simulink model "PX4HITLConnector"  (R2026a)
settings: Solver=VariableStepAuto
values from neighbouring files (symbols this model uses):
  gpsFreq = 25    [setUpHITLConnection.m]
  heartbeatFreq = 1    [setUpHITLConnection.m]
  SampleTime = 0.008    [setUpHITLConnection.m]
undefined symbols (not defined in the file or in its folder): controllerArmed, EngineCommandBus, Payload, ServosCommandBus
libraries: uavmavlinklib x7, simulink x4, px4MAVLinkBridgelib x2
settings Model: Creator=Usuario  LastModifiedBy=Usuario

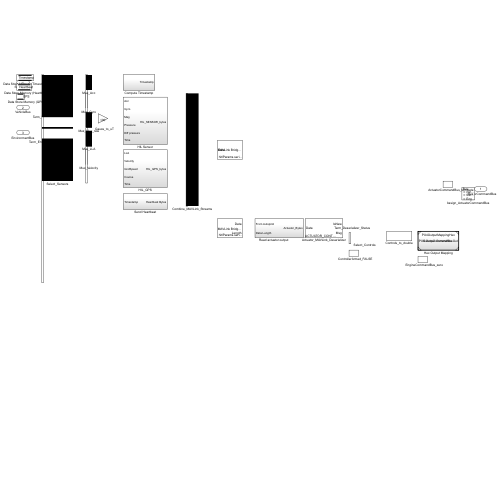
[thumbnail: Simulink's stored preview of the top-level diagram]
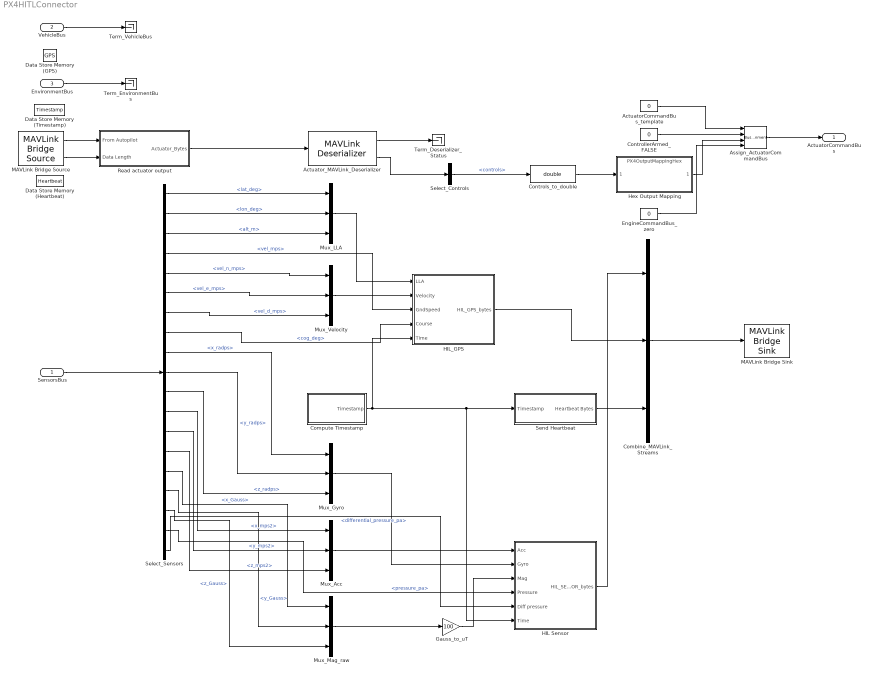
== system PX4HITLConnector ==
  SensorsBus : Inport  OutDataTypeStr=Bus: SensorsBus
  VehicleBus : Inport  Port=2  OutDataTypeStr=Bus: VehicleBus
  EnvironmentBus : Inport  Port=3  OutDataTypeStr=Bus: EnvironmentBus
  ActuatorCommandBus_template : Constant  Value=0  OutDataTypeStr=Bus: ActuatorCommandBus
  Actuator_MAVLink_Deserializer : uavmavlinklib/MAVLink Deserializer  dialectSource=Select from standard MAVLink dialects  dialect=common.xml  dialectCustom=common.xml  version=2  messageType=HIL_ACTUATOR_CONTROLS  inputDataLength=off  SystemIDFilter=off  systemID=1  ComponentIDFilter=off  componentID=1  queueMsg=off  queueMsgSize=50  dropNum=off
  Assign_ActuatorCommandBus : BusAssignment  AssignedSignals=controllerArmed,ServosCommandBus,EngineCommandBus
  Combine_MAVLink_Streams : Mux  Inputs=3
  Compute Timestamp : Subsystem  Priority=1
  ControllerArmed_FALSE : Constant  Value=0  OutDataTypeStr=double
  Controls_to_double : DataTypeConversion  OutDataTypeStr=double  SaturateOnIntegerOverflow=off  RndMeth=Floor
  Data Store Memory (GPS) : DataStoreMemory  DataStoreName=GPS  WriteAfterWriteMsg=warning  ShowAdditionalParam=off
  Data Store Memory (Heartbeat) : DataStoreMemory  DataStoreName=Heartbeat  WriteAfterWriteMsg=warning  ShowAdditionalParam=off
  Data Store Memory (Timestamp) : DataStoreMemory  DataStoreName=Timestamp  WriteAfterWriteMsg=warning  ShowAdditionalParam=off
  EngineCommandBus_zero : Constant  Value=0  OutDataTypeStr=Bus: EngineCommandBus
  Gauss_to_uT : Gain  Gain=100
  HIL Sensor : Subsystem  Priority=2
  HIL_GPS : Subsystem  Priority=3
  Hex Output Mapping : ModelReference  ModelNameDialog=PX4OutputMappingHex.slx  SimulationMode=Normal  ModelReferenceVersion=1.15
  MAVLink Bridge Sink : px4MAVLinkBridgelib/MAVLink Bridge Sink  PixhawkSerialPorttemp=Specify manually  PixhawkSerialPortManually=hitlParams.serialPort  FieldTable={'UDP', '127.0.0.1', '14550'}
  MAVLink Bridge Source : px4MAVLinkBridgelib/MAVLink Bridge Source  PixhawkSerialPorttemp=Specify manually  PixhawkSerialPortManually=hitlParams.serialPort  dataLength=1024  FieldTable={'UDP', '127.0.0.1', '14550'}  SampleTime=SampleTime
  Mux_Acc : Mux  Inputs=3
  Mux_Gyro : Mux  Inputs=3
  Mux_LLA : Mux  Inputs=3
  Mux_Mag_raw : Mux  Inputs=3
  Mux_Velocity : Mux  Inputs=3
  Read actuator output : Subsystem
  Select_Controls : BusSelector  OutputSignals=Payload.controls
  Select_Sensors : BusSelector  OutputSignals=GPSSensorBus.lat_deg,GPSSensorBus.lon_deg,GPSSensorBus.alt_m,GPSSensorBus.vel_mps,GPSSensorBus.vel_n_mps,GPSSensorBus.vel_e_mps,GPSSensorBus.vel_d_mps,GPSSensorBus.cog_deg,INSSensorBus.GyroSensorBus.x_radps,INSSensorBus.GyroSensorBus.y_radps,INSSensorBus.GyroSensorBus.z_radps,INSSensorBus.AccelSensorBus.x_mps2,INSSensorBus.AccelSensorBus.y_mps2,INSSensorBus.AccelSensorBus.z_mps2,INSSensorBus.MagSensorBus.x_Gauss,INSSensorBus.MagSensorBus.y_Gauss,INSSensorBus.MagSensorBus.z_Gauss,ADCSensorBus.BaroSensorBus.pressure_pa,ADCSensorBus.DiffPressureSensorBus.differential_pressure_pa
  Send Heartbeat : Subsystem  Priority=4
  Term_Deserializer_Status : Terminator
  Term_EnvironmentBus : Terminator
  Term_VehicleBus : Terminator
  ActuatorCommandBus : Outport  OutDataTypeStr=Bus: ActuatorCommandBus
  wires:
  Select_Sensors/18 -> HIL Sensor/4(Pressure)  "<pressure_pa>"
  Select_Sensors/1 -> Mux_LLA/1  "<lat_deg>"
  HIL_GPS/1(HIL_GPS_bytes) -> Combine_MAVLink_Streams/2
  Actuator_MAVLink_Deserializer/1 -> Term_Deserializer_Status/1
  VehicleBus/1 -> Term_VehicleBus/1
  MAVLink Bridge Source/2 -> Read actuator output/2(Data Length)
  Read actuator output/1(Actuator_Bytes) -> Actuator_MAVLink_Deserializer/1
  Mux_Mag_raw/1 -> Gauss_to_uT/1
  SensorsBus/1 -> Select_Sensors/1
  EnvironmentBus/1 -> Term_EnvironmentBus/1
  MAVLink Bridge Source/1 -> Read actuator output/1(From Autopilot)
  Select_Sensors/2 -> Mux_LLA/2  "<lon_deg>"
  Mux_Acc/1 -> HIL Sensor/1(Acc)
  Select_Sensors/3 -> Mux_LLA/3  "<alt_m>"
  Mux_Gyro/1 -> HIL Sensor/2(Gyro)
  Actuator_MAVLink_Deserializer/2 -> Select_Controls/1
  Select_Sensors/4 -> HIL_GPS/3(GndSpeed)  "<vel_mps>"
  Select_Sensors/5 -> Mux_Velocity/1  "<vel_n_mps>"
  Select_Sensors/11 -> Mux_Gyro/3  "<z_radps>"
  Select_Sensors/6 -> Mux_Velocity/2  "<vel_e_mps>"
  Select_Sensors/7 -> Mux_Velocity/3  "<vel_d_mps>"
  Mux_Velocity/1 -> HIL_GPS/2(Velocity)
  Select_Sensors/8 -> HIL_GPS/4(Course)  "<cog_deg>"
  HIL Sensor/1(HIL_SENSOR_bytes) -> Combine_MAVLink_Streams/1
  Select_Sensors/9 -> Mux_Gyro/1  "<x_radps>"
  ActuatorCommandBus_template/1 -> Assign_ActuatorCommandBus/1
  Select_Sensors/10 -> Mux_Gyro/2  "<y_radps>"
  Select_Sensors/12 -> Mux_Acc/1  "<x_mps2>"
  Select_Sensors/13 -> Mux_Acc/2  "<y_mps2>"
  Select_Sensors/14 -> Mux_Acc/3  "<z_mps2>"
  Select_Sensors/15 -> Mux_Mag_raw/1  "<x_Gauss>"
  Select_Sensors/16 -> Mux_Mag_raw/2  "<y_Gauss>"
  Select_Sensors/17 -> Mux_Mag_raw/3  "<z_Gauss>"
  Select_Sensors/19 -> HIL Sensor/5(Diff pressure)  "<differential_pressure_pa>"
  Mux_LLA/1 -> HIL_GPS/1(LLA)
  Compute Timestamp/1(Timestamp) -> Send Heartbeat/1(Timestamp), HIL Sensor/6(Time), HIL_GPS/5(Time)
  Controls_to_double/1 -> Hex Output Mapping/1
  Select_Controls/1 -> Controls_to_double/1  "<controls>"
  Gauss_to_uT/1 -> HIL Sensor/3(Mag)
  Combine_MAVLink_Streams/1 -> MAVLink Bridge Sink/1
  Send Heartbeat/1(Heartbeat Bytes) -> Combine_MAVLink_Streams/3
  ControllerArmed_FALSE/1 -> Assign_ActuatorCommandBus/2
  Hex Output Mapping/1 -> Assign_ActuatorCommandBus/3
  EngineCommandBus_zero/1 -> Assign_ActuatorCommandBus/4
  Assign_ActuatorCommandBus/1 -> ActuatorCommandBus/1

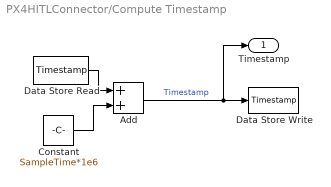
== system PX4HITLConnector/Compute Timestamp ==
  Add : Sum
  Constant : Constant  Value=SampleTime*1e6  OutDataTypeStr=uint64  SampleTime=SampleTime
  Data Store Read : DataStoreRead  DataStoreName=Timestamp  SampleTime=SampleTime  IndexOptions=Index vector (dialog)  Indices=1  OutputSizes=1
  Data Store Write : DataStoreWrite  DataStoreName=Timestamp  SampleTime=SampleTime  IndexOptions=Index vector (dialog)  Indices=1  OutputSizes=1
  Timestamp : Outport
  wires:
  Constant/1 -> Add/2
  Add/1 -> Data Store Write/1, Timestamp/1  "Timestamp"
  Data Store Read/1 -> Add/1

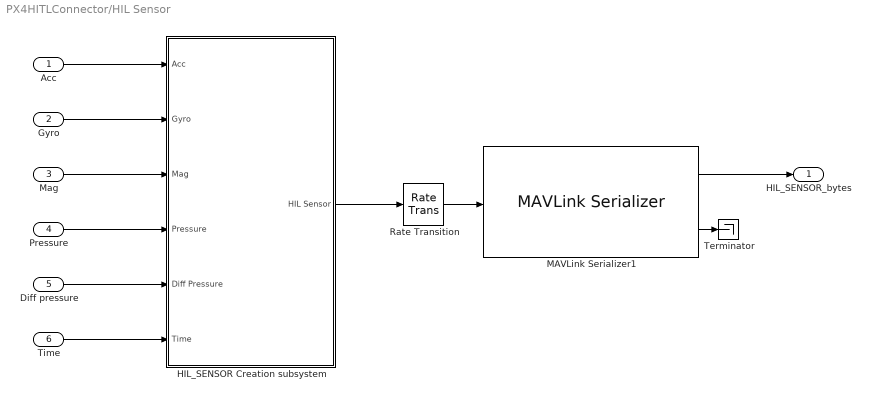
== system PX4HITLConnector/HIL Sensor ==
  Acc : Inport
  Gyro : Inport  Port=2
  Mag : Inport  Port=3
  Pressure : Inport  Port=4
  Diff pressure : Inport  Port=5
  Time : Inport  Port=6
  HIL_SENSOR Creation subsystem : Subsystem
  MAVLink Serializer1 : uavmavlinklib/MAVLink Serializer  dialectSource=Select from standard MAVLink dialects  dialect=common.xml  dialectCustom=common.xml  version=2  messageType=HIL_SENSOR
  Rate Transition : RateTransition  OutPortSampleTime=SampleTime
  Terminator : Terminator
  HIL_SENSOR_bytes : Outport
  wires:
  Time/1 -> HIL_SENSOR Creation subsystem/6(Time)
  HIL_SENSOR Creation subsystem/1(HIL Sensor) -> Rate Transition/1
  MAVLink Serializer1/1 -> HIL_SENSOR_bytes/1
  MAVLink Serializer1/2 -> Terminator/1
  Rate Transition/1 -> MAVLink Serializer1/1
  Diff pressure/1 -> HIL_SENSOR Creation subsystem/5(Diff Pressure)
  Pressure/1 -> HIL_SENSOR Creation subsystem/4(Pressure)
  Mag/1 -> HIL_SENSOR Creation subsystem/3(Mag)
  Gyro/1 -> HIL_SENSOR Creation subsystem/2(Gyro)
  Acc/1 -> HIL_SENSOR Creation subsystem/1(Acc)

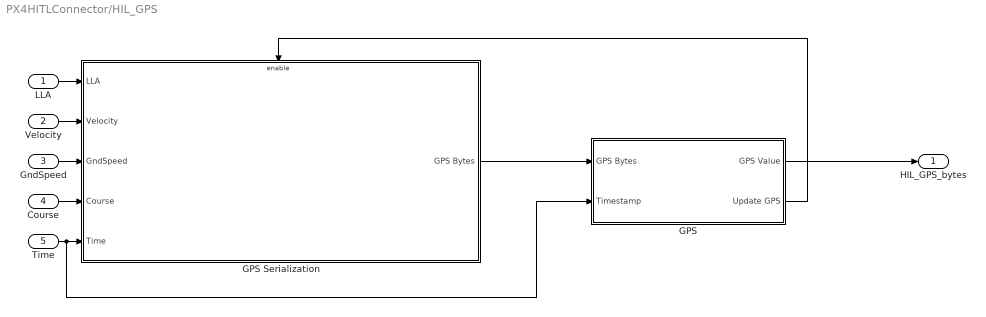
== system PX4HITLConnector/HIL_GPS ==
  LLA : Inport
  Velocity : Inport  Port=2
  GndSpeed : Inport  Port=3
  Course : Inport  Port=4
  Time : Inport  Port=5
  GPS : Subsystem
  GPS Serialization : Subsystem
  HIL_GPS_bytes : Outport
  wires:
  GPS/2(Update GPS) -> GPS Serialization/Enable
  GPS/1(GPS Value) -> HIL_GPS_bytes/1
  GPS Serialization/1(GPS Bytes) -> GPS/1(GPS Bytes)
  Time/1 -> GPS Serialization/5(Time), GPS/2(Timestamp)
  Course/1 -> GPS Serialization/4(Course)
  GndSpeed/1 -> GPS Serialization/3(GndSpeed)
  Velocity/1 -> GPS Serialization/2(Velocity)
  LLA/1 -> GPS Serialization/1(LLA)

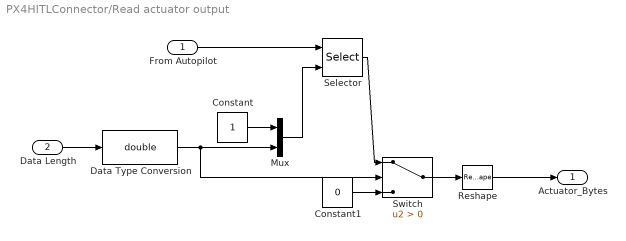
== system PX4HITLConnector/Read actuator output ==
  From Autopilot : Inport
  Data Length : Inport  Port=2
  Constant : Constant  SampleTime=SampleTime
  Constant1 : Constant  Value=0  OutDataTypeStr=uint8  SampleTime=SampleTime
  Data Type Conversion : DataTypeConversion  OutDataTypeStr=double  SaturateOnIntegerOverflow=off  RndMeth=Floor
  Mux : Mux  Inputs=2
  Reshape : Reshape
  Selector : Selector  InputPortWidth=MAVLink_Input_Read_Size  IndexOptions=Starting and ending indices (port)  Indices=[1 3]  OutputSizes=1
  Switch : Switch  Criteria=u2 > Threshold  SaturateOnIntegerOverflow=off  InputSameDT=off
  Actuator_Bytes : Outport
  wires:
  Constant1/1 -> Switch/3
  Reshape/1 -> Actuator_Bytes/1
  Data Type Conversion/1 -> Mux/2, Switch/2
  Selector/1 -> Switch/1
  Switch/1 -> Reshape/1
  From Autopilot/1 -> Selector/1
  Data Length/1 -> Data Type Conversion/1
  Constant/1 -> Mux/1
  Mux/1 -> Selector/2

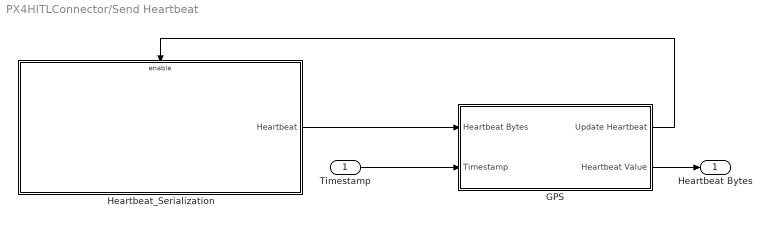
== system PX4HITLConnector/Send Heartbeat ==
  Timestamp : Inport
  GPS : Subsystem
  Heartbeat_Serialization : Subsystem
  Heartbeat Bytes : Outport
  wires:
  GPS/2(Heartbeat Value) -> Heartbeat Bytes/1
  GPS/1(Update Heartbeat) -> Heartbeat_Serialization/Enable
  Timestamp/1 -> GPS/2(Timestamp)
  Heartbeat_Serialization/1(Heartbeat) -> GPS/1(Heartbeat Bytes)

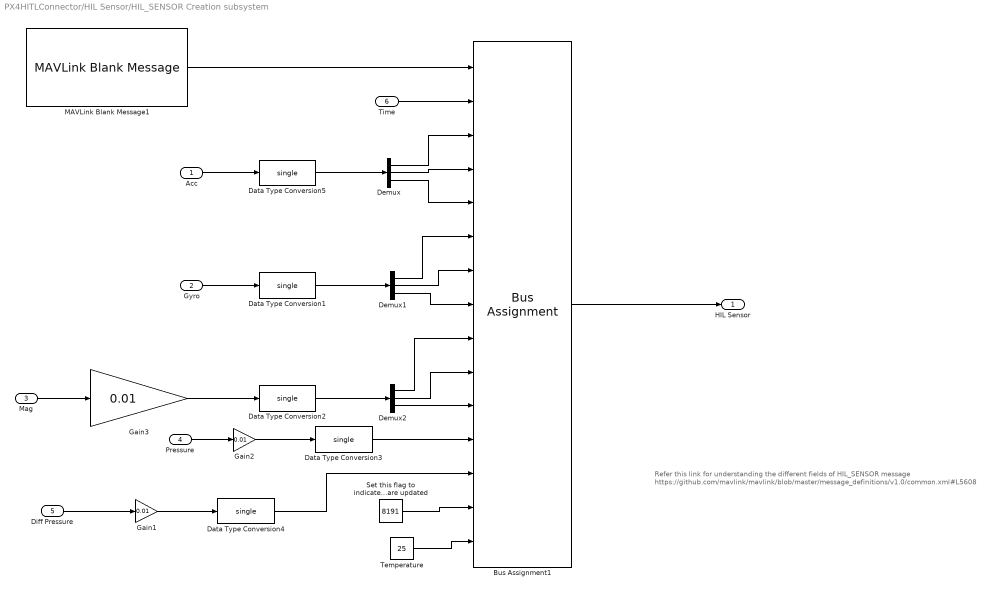
== system PX4HITLConnector/HIL Sensor/HIL_SENSOR Creation subsystem ==
  note: Refer this link for understanding the different fields of HIL_SENSOR message https://github.com/mavlink/mavlink/blob/master/message_definitions/v1.0/common.xml#L5608
  Acc : Inport
  Gyro : Inport  Port=2
  Mag : Inport  Port=3
  Pressure : Inport  Port=4
  Diff Pressure : Inport  Port=5
  Time : Inport  Port=6
  Bus Assignment1 : BusAssignment  AssignedSignals=Payload.time_usec,Payload.xacc,Payload.yacc,Payload.zacc,Payload.xgyro,Payload.ygyro,Payload.zgyro,Payload.xmag,Payload.ymag,Payload.zmag,Payload.abs_pressure,Payload.diff_pressure,Payload.fields_updated,Payload.temperature
  Data Type Conversion{1..5} (5 alike) : DataTypeConversion  OutDataTypeStr=single  SaturateOnIntegerOverflow=off  RndMeth=Floor
  Demux : Demux  Outputs=3
  Demux1 : Demux  Outputs=3
  Demux2 : Demux  Outputs=3
  Gain1 : Gain  Gain=0.01  OutDataTypeStr=single
  Gain2 : Gain  Gain=0.01  OutDataTypeStr=single
  Gain3 : Gain  Gain=0.01
  MAVLink Blank Message1 : uavmavlinklib/MAVLink Blank Message  dialectSource=Select from standard MAVLink dialects  dialect=common.xml  dialectCustom=common.xml  version=2  messageType=HIL_SENSOR  SystemID=2  ComponentID=51  SampleTime=-1
  Set this flag to indicate all flags are updated : Constant  Value=8191  OutDataTypeStr=Inherit: Inherit via back propagation  SampleTime=-1
  Temperature : Constant  Value=25  OutDataTypeStr=Inherit: Inherit via back propagation  SampleTime=-1
  HIL Sensor : Outport
  wires:
  Data Type Conversion4/1 -> Bus Assignment1/13
  Gain1/1 -> Data Type Conversion4/1
  Diff Pressure/1 -> Gain1/1
  Temperature/1 -> Bus Assignment1/15
  Gain2/1 -> Data Type Conversion3/1
  Time/1 -> Bus Assignment1/2
  Pressure/1 -> Gain2/1
  Set this flag to indicate all flags are updated/1 -> Bus Assignment1/14
  Gain3/1 -> Data Type Conversion2/1
  Data Type Conversion3/1 -> Bus Assignment1/12
  Acc/1 -> Data Type Conversion5/1
  Demux1/2 -> Bus Assignment1/7
  Demux/2 -> Bus Assignment1/4
  Demux2/1 -> Bus Assignment1/9
  MAVLink Blank Message1/1 -> Bus Assignment1/1
  Demux/1 -> Bus Assignment1/3
  Data Type Conversion5/1 -> Demux/1
  Demux2/3 -> Bus Assignment1/11
  Demux2/2 -> Bus Assignment1/10
  Demux/3 -> Bus Assignment1/5
  Bus Assignment1/1 -> HIL Sensor/1
  Gyro/1 -> Data Type Conversion1/1
  Data Type Conversion1/1 -> Demux1/1
  Demux1/3 -> Bus Assignment1/8
  Mag/1 -> Gain3/1
  Demux1/1 -> Bus Assignment1/6
  Data Type Conversion2/1 -> Demux2/1

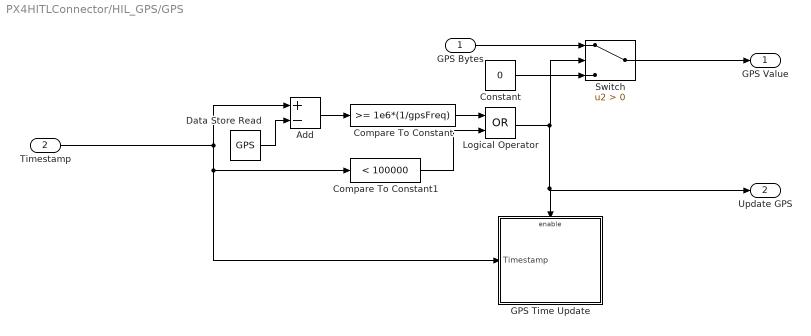
== system PX4HITLConnector/HIL_GPS/GPS ==
  GPS Bytes : Inport
  Timestamp : Inport  Port=2
  Add : Sum  Inputs=+-
  Compare To Constant : simulink/Logic and Bit Operations/Compare To Constant  relop=>=  const=1e6*(1/gpsFreq)  OutDataTypeStr=uint8
  Compare To Constant1 : simulink/Logic and Bit Operations/Compare To Constant  relop=<  const=100000  OutDataTypeStr=boolean
  Constant : Constant  Value=0  OutDataTypeStr=uint8  SampleTime=SampleTime
  Data Store Read : DataStoreRead  DataStoreName=GPS  SampleTime=SampleTime  IndexOptions=Index vector (dialog)  Indices=1  OutputSizes=1
  GPS Time Update : Subsystem
  Logical Operator : Logic  Operator=OR  AllPortsSameDT=off  OutDataTypeStr=boolean
  Switch : Switch  Criteria=u2 > Threshold  SaturateOnIntegerOverflow=off  InputSameDT=off
  GPS Value : Outport
  Update GPS : Outport  Port=2
  wires:
  Compare To Constant1/1 -> Logical Operator/2
  Logical Operator/1 -> Switch/2, Update GPS/1, GPS Time Update/Enable
  Compare To Constant/1 -> Logical Operator/1
  Switch/1 -> GPS Value/1
  Constant/1 -> Switch/3
  GPS Bytes/1 -> Switch/1
  Add/1 -> Compare To Constant/1
  Data Store Read/1 -> Add/2
  Timestamp/1 -> Add/1, Compare To Constant1/1, GPS Time Update/1(Timestamp)

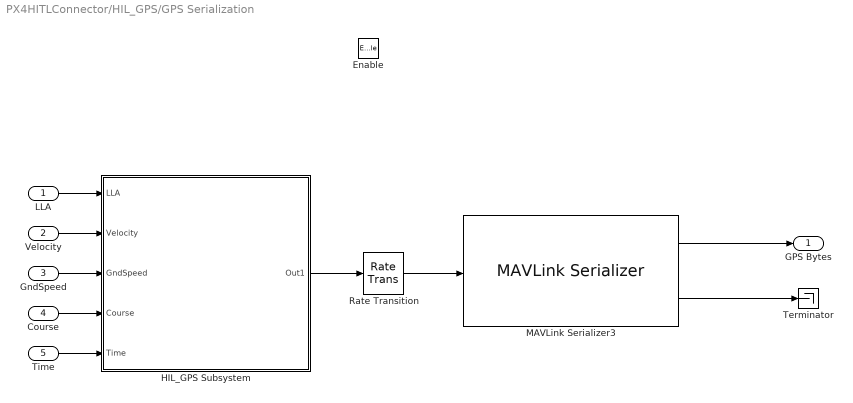
== system PX4HITLConnector/HIL_GPS/GPS Serialization ==
  LLA : Inport
  Velocity : Inport  Port=2
  GndSpeed : Inport  Port=3
  Course : Inport  Port=4
  Time : Inport  Port=5
  Enable : EnablePort
  HIL_GPS Subsystem : Subsystem
  MAVLink Serializer3 : uavmavlinklib/MAVLink Serializer  dialectSource=Select from standard MAVLink dialects  dialect=common.xml  dialectCustom=common.xml  version=2  messageType=HIL_GPS
  Rate Transition : RateTransition  OutPortSampleTime=SampleTime
  Terminator : Terminator
  GPS Bytes : Outport
  wires:
  GndSpeed/1 -> HIL_GPS Subsystem/3(GndSpeed)
  Time/1 -> HIL_GPS Subsystem/5(Time)
  Course/1 -> HIL_GPS Subsystem/4(Course)
  LLA/1 -> HIL_GPS Subsystem/1(LLA)
  HIL_GPS Subsystem/1(Out1) -> Rate Transition/1
  MAVLink Serializer3/2 -> Terminator/1
  Rate Transition/1 -> MAVLink Serializer3/1
  Velocity/1 -> HIL_GPS Subsystem/2(Velocity)
  MAVLink Serializer3/1 -> GPS Bytes/1

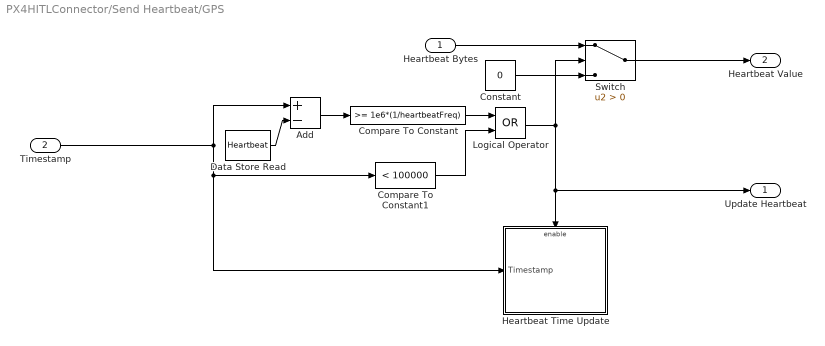
== system PX4HITLConnector/Send Heartbeat/GPS ==
  Heartbeat Bytes : Inport
  Timestamp : Inport  Port=2
  Add : Sum  Inputs=+-
  Compare To Constant : simulink/Logic and Bit Operations/Compare To Constant  relop=>=  const=1e6*(1/heartbeatFreq)  OutDataTypeStr=uint8
  Compare To Constant1 : simulink/Logic and Bit Operations/Compare To Constant  relop=<  const=100000  OutDataTypeStr=boolean
  Constant : Constant  Value=0  OutDataTypeStr=uint8  SampleTime=SampleTime
  Data Store Read : DataStoreRead  DataStoreName=Heartbeat  SampleTime=SampleTime  IndexOptions=Index vector (dialog)  Indices=1  OutputSizes=1
  Heartbeat Time Update : Subsystem
  Logical Operator : Logic  Operator=OR  AllPortsSameDT=off  OutDataTypeStr=boolean
  Switch : Switch  Criteria=u2 > Threshold  SaturateOnIntegerOverflow=off  InputSameDT=off
  Update Heartbeat : Outport
  Heartbeat Value : Outport  Port=2
  wires:
  Logical Operator/1 -> Heartbeat Time Update/Enable, Update Heartbeat/1, Switch/2
  Compare To Constant/1 -> Logical Operator/1
  Compare To Constant1/1 -> Logical Operator/2
  Switch/1 -> Heartbeat Value/1
  Constant/1 -> Switch/3
  Heartbeat Bytes/1 -> Switch/1
  Add/1 -> Compare To Constant/1
  Data Store Read/1 -> Add/2
  Timestamp/1 -> Add/1, Compare To Constant1/1, Heartbeat Time Update/1(Timestamp)

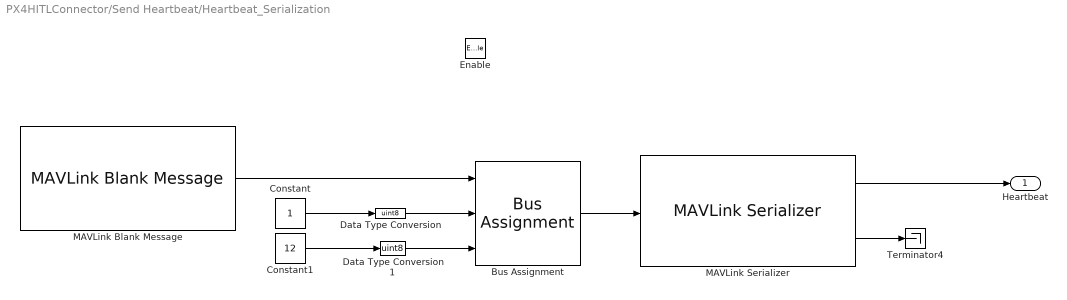
== system PX4HITLConnector/Send Heartbeat/Heartbeat_Serialization ==
  Enable : EnablePort
  Bus Assignment : BusAssignment  AssignedSignals=Payload.autopilot,Payload.type
  Constant : Constant  SampleTime=-1
  Constant1 : Constant  Value=12  SampleTime=-1
  Data Type Conversion : DataTypeConversion  OutDataTypeStr=uint8  SaturateOnIntegerOverflow=off  RndMeth=Floor
  Data Type Conversion1 : DataTypeConversion  OutDataTypeStr=uint8  SaturateOnIntegerOverflow=off  RndMeth=Floor
  MAVLink Blank Message : uavmavlinklib/MAVLink Blank Message  dialectSource=Select from standard MAVLink dialects  dialect=common.xml  dialectCustom=common.xml  version=2  messageType=HEARTBEAT  SystemID=2  ComponentID=51  SampleTime=SampleTime
  MAVLink Serializer : uavmavlinklib/MAVLink Serializer  dialectSource=Select from standard MAVLink dialects  dialect=common.xml  dialectCustom=common.xml  version=2  messageType=HEARTBEAT
  Terminator4 : Terminator
  Heartbeat : Outport
  wires:
  MAVLink Serializer/1 -> Heartbeat/1
  MAVLink Blank Message/1 -> Bus Assignment/1
  Data Type Conversion/1 -> Bus Assignment/2
  MAVLink Serializer/2 -> Terminator4/1
  Bus Assignment/1 -> MAVLink Serializer/1
  Constant1/1 -> Data Type Conversion1/1
  Constant/1 -> Data Type Conversion/1
  Data Type Conversion1/1 -> Bus Assignment/3

== system PX4HITLConnector/HIL_GPS/GPS/GPS Time Update ==
  Timestamp : Inport
  Enable : EnablePort
  Update GPS Time : DataStoreWrite  DataStoreName=GPS  IndexOptions=Index vector (dialog)  Indices=1  OutputSizes=1
  wires:
  Timestamp/1 -> Update GPS Time/1

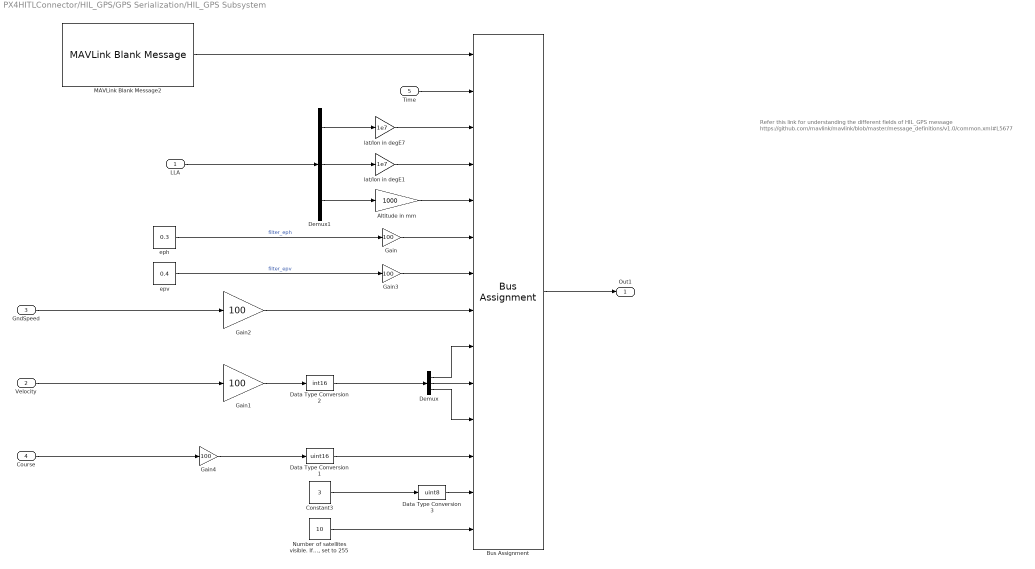
== system PX4HITLConnector/HIL_GPS/GPS Serialization/HIL_GPS Subsystem ==
  note: Refer this link for understanding the different fields of HIL_GPS message https://github.com/mavlink/mavlink/blob/master/message_definitions/v1.0/common.xml#L5677
  LLA : Inport
  Velocity : Inport  Port=2
  GndSpeed : Inport  Port=3
  Course : Inport  Port=4
  Time : Inport  Port=5
  Altitude in mm : Gain  Gain=1000  OutDataTypeStr=Inherit: Inherit via back propagation
  Bus Assignment : BusAssignment  AssignedSignals=Payload.time_usec,Payload.lat,Payload.lon,Payload.alt,Payload.eph,Payload.epv,Payload.vel,Payload.vn,Payload.ve,Payload.vd,Payload.cog,Payload.fix_type,Payload.satellites_visible
  Constant3 : Constant  Value=3  OutDataTypeStr=Inherit: Inherit via back propagation  SampleTime=-1
  Data Type Conversion1 : DataTypeConversion  OutDataTypeStr=uint16  SaturateOnIntegerOverflow=off  RndMeth=Floor
  Data Type Conversion2 : DataTypeConversion  OutDataTypeStr=int16  SaturateOnIntegerOverflow=off  RndMeth=Floor
  Data Type Conversion3 : DataTypeConversion  OutDataTypeStr=uint8  SaturateOnIntegerOverflow=off  RndMeth=Floor
  Demux : Demux  Outputs=3
  Demux1 : Demux  Outputs=3
  Gain : Gain  Gain=100  OutDataTypeStr=Inherit: Inherit via back propagation
  Gain1 : Gain  Gain=100
  Gain2 : Gain  Gain=100  OutDataTypeStr=uint16
  Gain3 : Gain  Gain=100  OutDataTypeStr=Inherit: Inherit via back propagation
  Gain4 : Gain  Gain=100
  MAVLink Blank Message2 : uavmavlinklib/MAVLink Blank Message  dialectSource=Select from standard MAVLink dialects  dialect=common.xml  dialectCustom=common.xml  version=2  messageType=HIL_GPS  SystemID=2  ComponentID=51  SampleTime=-1
  "Number of satellites visible. If unknown, set to 255" : Constant  Value=10  OutDataTypeStr=Inherit: Inherit via back propagation  SampleTime=-1
  eph : Constant  Value=0.3  SampleTime=-1
  epv : Constant  Value=0.4  SampleTime=-1
  lat/lon in degE1 : Gain  Gain=1e7  OutDataTypeStr=Inherit: Inherit via back propagation
  lat/lon in degE7 : Gain  Gain=1e7  OutDataTypeStr=Inherit: Inherit via back propagation
  Out1 : Outport
  wires:
  "Number of satellites visible. If unknown, set to 255"/1 -> Bus Assignment/14
  Constant3/1 -> Data Type Conversion3/1
  Bus Assignment/1 -> Out1/1
  LLA/1 -> Demux1/1
  Time/1 -> Bus Assignment/2
  Gain4/1 -> Data Type Conversion1/1
  Data Type Conversion3/1 -> Bus Assignment/13
  epv/1 -> Gain3/1  "filter_epv"
  eph/1 -> Gain/1  "filter_eph"
  Data Type Conversion1/1 -> Bus Assignment/12
  Course/1 -> Gain4/1
  Velocity/1 -> Gain1/1
  GndSpeed/1 -> Gain2/1
  Gain3/1 -> Bus Assignment/7
  Gain/1 -> Bus Assignment/6
  Demux/2 -> Bus Assignment/10
  Data Type Conversion2/1 -> Demux/1
  Altitude in mm/1 -> Bus Assignment/5
  lat/lon in degE1/1 -> Bus Assignment/4
  Demux/1 -> Bus Assignment/9
  Demux1/2 -> lat/lon in degE1/1
  Demux1/3 -> Altitude in mm/1
  Gain1/1 -> Data Type Conversion2/1
  MAVLink Blank Message2/1 -> Bus Assignment/1
  Demux/3 -> Bus Assignment/11
  Demux1/1 -> lat/lon in degE7/1
  lat/lon in degE7/1 -> Bus Assignment/3
  Gain2/1 -> Bus Assignment/8

== system PX4HITLConnector/Send Heartbeat/GPS/Heartbeat Time Update ==
  Timestamp : Inport
  Enable : EnablePort
  Update Heartbeat Time : DataStoreWrite  DataStoreName=Heartbeat  IndexOptions=Index vector (dialog)  Indices=1  OutputSizes=1
  wires:
  Timestamp/1 -> Update Heartbeat Time/1
